simulink model "projectttt"  (R2021a)
settings: Solver=VariableStepAuto  StartTime=0.0  StopTime=3600*3  RelTol=1e-3
undefined symbols (not defined in the file): Ion, Lithium
libraries: spsBatteryLib x1, spsCurrentMeasurementLib x1, spsDCMachineLib x1, spspowerguiLib x1
settings Model: Creator=User  LastModifiedBy=User

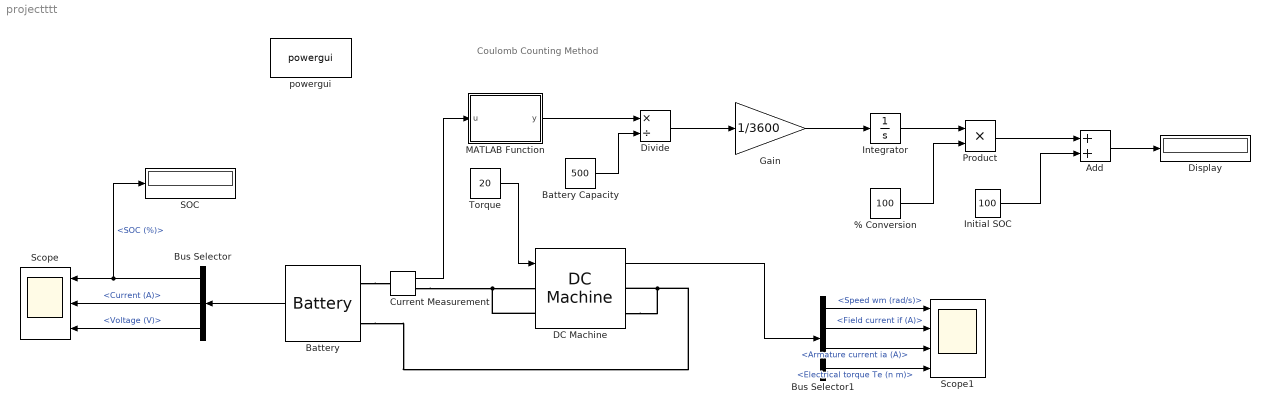
== system projectttt ==
  note: Coulomb Counting Method
  "% Conversion " : Constant  Value=100
  Add : Sum
  "Battery " : spsBatteryLib/Battery  BatType=Lithium-Ion  ShowTempParam=off  ThermalPreset=no  ShowAgeParam=off  NomV=12  NomQ=500  SOC=100  Batt_Tr=30  PresetModel=on  MaxQ=500  MinV=9  FullV=13.9678  Dis_rate=217.3913  R=0.00024  Normal_OP=452.1739  expZone="[12.9646      24.5652]"  current=[6.5 13 32.5]  Units=Time  Tci=20  NomT=20  T2=-30  MaxQ2=4.8  FullV2=7.1  Normal_OP2=5.655  expZone2="[6.58           1]"  Rca=0.6  ti=2000  Dp=0  Neq0=0  Tsim=1e6  Ta1=25  Qeol=5.4*0.9  Reol=0.013333*1.2  Char_age=[2.3478, 3]  Dis_age=[2.3478, 10]  N1=1500  N2=10500  N3=1000  N4=1400  Ta2=45  N5=950
  Battery Capacity : Constant  Value=500
  Bus Selector : BusSelector  OutputSignals=SOC (%),Current (A),Voltage (V)
  Bus Selector1 : BusSelector  OutputSignals=Speed wm (rad/s),Field current if (A),Armature current ia (A),Electrical torque Te (n m)
  Current Measurement : spsCurrentMeasurementLib/Current Measurement  PhasorSimulation=off  OutputType=Complex  PSBequivalent=0
  "DC Machine " : spsDCMachineLib/DC Machine  PresetModel=01: 5HP 240V 1750RPM Field:300V  MechanicalLoad=Torque TL  FieldType=Wound  ShowDetailedParameters=on  MeasurementBus=off  RLa=[2.581 0.028]  RLf=[281.3 156]  Laf=0.9483  MachineConstant=Torque constant (N.m/A)  Ke=1.8  Kt=1.8  J=0.02215  Bm=0.002953  Tf=0.5161  w0=1  Ifinit=0  TsPowergui=0  TsBlock=-1
  Display : Display
  Divide : Product  Inputs=*/
  Gain : Gain  Gain=1/3600
  Initial SOC : Constant  Value=100
  "Integrator " : Integrator
  MATLAB Function : MATLAB Function  TreatAsAtomicUnit=on
  Product : Product
  SOC : Display
  Scope : Scope  NumInputPorts=3
  Scope1 : Scope  NumInputPorts=4
  Torque : Constant  Value=20
  powergui : spspowerguiLib/powergui  Priority=1  SimulationMode=Continuous  SampleTime=50e-6  frequency=60  Iterations=50  frequencyindice=0  Pbase=100e6  ErrMax=1e-4  UnitsV=kV  UnitsW=MW  buscounter=0  FunctionMessages=off  echomessages=off  EnableUseOfTLC=off  CurrentSourceSwitches=off  DisableSnubberDevices=off  DisableRonSwitches=off  DisableVfSwitches=off  DisplayEquations=off  AutomaticDiscreteSolvers=off  SolverType=Tustin/Backward Euler (TBE)  Interpol=off  ExternalGateDelay=off  methode=off  Ts=100  x0status=blocks  SPID=on  SwTol=0  HookPort=off  NonlinearTolerance=1e-4  nMaxIteration=100  ContinueOnMaxIteration=off  RestoreLinks=warning  ResistiveCurrentMeasurement=off  Frange=[0:2:500]  Ylog=off  Xlog=on  ShowGrid=off  save=off  variable=ZData  structure=0  ZoomFFT=off  StartTime=0.0  cycles=1  DisplayStyle=1  fundamental=60  FreqAxis=off  MaxFrequency=1000  frequencyindicesteady=1  RmsSteady=1  display=off
  wires:
  Torque/1 -> "DC Machine "/1
  "Battery "/1 -> Bus Selector/1
  Bus Selector/3 -> Scope/3  "<Voltage (V)>"
  Bus Selector/2 -> Scope/2  "<Current (A)>"
  Bus Selector/1 -> SOC/1, Scope/1  "<SOC (%)>"
  Current Measurement/1 -> MATLAB Function/1(u)
  MATLAB Function/1(y) -> Divide/1
  Battery Capacity/1 -> Divide/2
  Divide/1 -> Gain/1
  Gain/1 -> "Integrator "/1
  "Integrator "/1 -> Product/1
  "% Conversion "/1 -> Product/2
  Product/1 -> Add/1
  Initial SOC/1 -> Add/2
  Add/1 -> Display/1
  "DC Machine "/1 -> Bus Selector1/1
  Bus Selector1/1 -> Scope1/1  "<Speed wm (rad/s)>"
  Bus Selector1/2 -> Scope1/2  "<Field current if (A)>"
  Bus Selector1/3 -> Scope1/3  "<Armature current ia (A)>"
  Bus Selector1/4 -> Scope1/4  "<Electrical torque Te (n m)>"
  connections:
  "Battery "/LConn2 -- "DC Machine "/RConn2 -- "DC Machine "/RConn1
  "Battery "/LConn1 -- Current Measurement/LConn1
  Current Measurement/RConn1 -- "DC Machine "/LConn2 -- "DC Machine "/LConn1

== matlab function projectttt/MATLAB Function ==
  data: u input; y output
function y = fcn(u)

y = -u;
